simulink model "motor"  (R2019b)
settings: Solver=VariableStepAuto  StartTime=0.0  StopTime=10.0  RelTol=1e-3
settings Model: Creator=Kyungpyo  LastModifiedBy=Kyungpyo

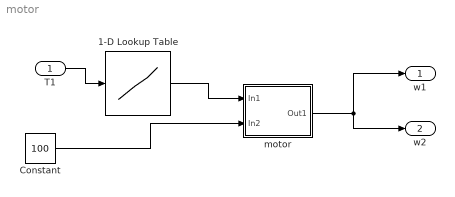
== system motor ==
  T1 : Inport
  1-D Lookup Table : Lookup_n-D  NumberOfTableDimensions=1  BreakpointsForDimension1=[-5:5]  Table=tanh([-5:5])  InternalRulePriority=Speed  RndMeth=Simplest  InputSameDT=on
  Constant : Constant  Value=100
  motor : Subsystem
  w1 : Outport
  w2 : Outport  Port=2
  wires:
  motor/1(Out1) -> w1/1, w2/1
  Constant/1 -> motor/2(In2)
  T1/1 -> 1-D Lookup Table/1
  1-D Lookup Table/1 -> motor/1(In1)

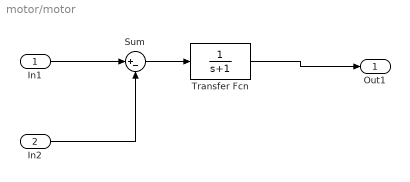
== system motor/motor ==
  In1 : Inport
  In2 : Inport  Port=2
  Sum : Sum  Inputs=|+-
  Transfer Fcn : TransferFcn  Denominator=[1 1]
  Out1 : Outport
  wires:
  Sum/1 -> Transfer Fcn/1
  Transfer Fcn/1 -> Out1/1
  In2/1 -> Sum/2
  In1/1 -> Sum/1
